simulink model "flightController"  (R2021a)
settings: Solver=ode3  StartTime=0  StopTime=TFinal  FixedStep=Ts  RelTol=1e-3  EnableMultiTasking=on
undefined symbols (not defined in the file): A, B, Controller, DiscIntNeverNeededParam, g, K, KLQI, KLQR, linsys, Ts, Vehicle
settings Model: Creator=The MathWorks, Inc.  LastModifiedBy=John
settings SolverCC: AlgebraicLoopSolver=TrustRegion  MinimalZcImpactIntegration=on
settings DataIOCC: LimitDataPoints=on  SaveFormat=Array  ReturnWorkspaceOutputs=off
settings OptimizationCC: BlockReduction=off  DefaultParameterBehavior=Inlined  BufferReuse=off  PassReuseOutputArgsThreshold=0
settings DebuggingCC: AlgebraicLoopMsg=none  ParameterPrecisionLossMsg=none  ParameterTunabilityLossMsg=error  UnconnectedInputMsg=none  UnconnectedOutputMsg=none  UnconnectedLineMsg=none  BusObjectLabelMismatch=error  SFUnexpectedBacktrackingDiag=warning  SFNoUnconditionalDefaultTransitionDiag=warning  SFExecutionAtInitializationDiag=none  SFMachineParentedDataDiag=warning  ArithmeticOperatorsInVariantConditions=warning
settings HardwareCC: ProdBitPerPointer=32  ProdBitPerSizeT=32  ProdBitPerPtrDiffT=32  ProdLargestAtomicInteger=Long  ProdWordSize=32  ProdHWDeviceType=ARM Compatible->ARM 9
settings ModelReferenceCC: ModelReferenceNumInstancesAllowed=Single  PropagateSignalLabelsOutOfModel=off
settings SFSimCC: SimUseLocalCustomCode=off  CustomCodeUndefinedFunction=UseInterfaceOnly
settings RTWCC: Description=Generic Real-Time Target  GenerateReport=on  RTWUseLocalCustomCode=off  LaunchReport=on
settings CodeAppCC: ForceParamTrailComments=on  MaxIdLength=63  OperatorAnnotations=on  StateflowObjectComments=on  MATLABSourceComments=on
settings GRTTargetCC: TargetLangStandard=C89/C90 (ANSI)
settings ConfigComp: CovMetricSettings=dw  CovSaveCumulativeToWorkspaceVar=on  CovSaveSingleToWorkspaceVar=on  CovExternalEMLEnable=off  CovSFcnEnable=off

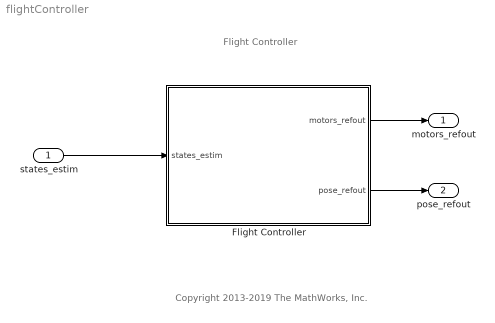
== system flightController ==
  note: Flight Controller
  note: Copyright 2013-2019 The MathWorks, Inc.
  states_estim : Inport  OutDataTypeStr=Bus: statesEstim_t  BusOutputAsStruct=on
  Flight Controller : Subsystem
  motors_refout : Outport  VectorParamsAs1DForOutWhenUnconnected=off
  pose_refout : Outport  Port=2  VectorParamsAs1DForOutWhenUnconnected=off
  wires:
  states_estim/1 -> Flight Controller/1(states_estim)
  Flight Controller/2(pose_refout) -> pose_refout/1
  Flight Controller/1(motors_refout) -> motors_refout/1

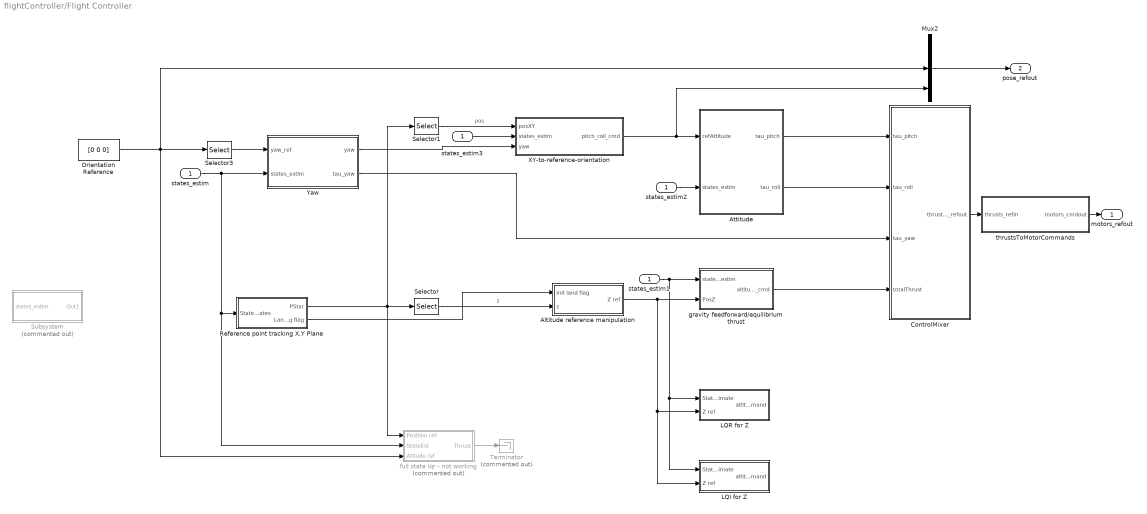
== system flightController/Flight Controller ==
  states_estim : Inport
  Altitude reference manipulation : Subsystem
  Attitude : Subsystem
  ControlMixer : Subsystem
  LQI for Z : Subsystem
  LQR for Z : Subsystem
  Mux2 : Mux  Inputs=3
  Orientation Reference : Constant  Value=[0 0 0]  OutDataTypeStr=single
  Reference point tracking X,Y Plane : Subsystem
  Selector : Selector  InputPortWidth=3  IndexOptions=Index vector (dialog)  Indices=3  OutputSizes=1
  Selector1 : Selector  InputPortWidth=3  IndexOptions=Index vector (dialog)  Indices=[1 2]  OutputSizes=1
  Selector3 : Selector  InputPortWidth=3  IndexOptions=Index vector (dialog)  Indices=1  OutputSizes=1
  Subsystem : Subsystem  Commented=on
  Terminator : Terminator  Commented=on
  XY-to-reference-orientation : Subsystem
  Yaw : Subsystem
  full state lqr - not working : Subsystem  Commented=on
  gravity feedforward/equilibrium thrust : Subsystem
  states_estim1 : InportShadow
  states_estim2 : InportShadow
  states_estim3 : InportShadow
  thrustsToMotorCommands : Subsystem
  motors_refout : Outport  VectorParamsAs1DForOutWhenUnconnected=off
  pose_refout : Outport  Port=2  VectorParamsAs1DForOutWhenUnconnected=off
  wires:
  thrustsToMotorCommands/1(motors_cmdout) -> motors_refout/1
  Selector3/1 -> Yaw/1(yaw_ref)
  Selector1/1 -> XY-to-reference-orientation/1(posXY)  "pos"
  ControlMixer/1(thrusts_refout) -> thrustsToMotorCommands/1(thrusts_refin)
  XY-to-reference-orientation/1(pitch_roll_cmd) -> Mux2/3, Attitude/1(refAttitude)
  Yaw/1(yaw) -> XY-to-reference-orientation/3(yaw)
  Mux2/1 -> pose_refout/1
  Attitude/1(tau_pitch) -> ControlMixer/1(tau_pitch)
  Attitude/2(tau_roll) -> ControlMixer/2(tau_roll)
  Yaw/2(tau_yaw) -> ControlMixer/3(tau_yaw)
  states_estim1/1 -> gravity feedforward/equilibrium thrust/1(states_estim), LQI for Z/1(State estimate), LQR for Z/1(State Estimate)
  states_estim2/1 -> Attitude/2(states_estim)
  states_estim3/1 -> XY-to-reference-orientation/2(states_estim)
  Orientation Reference/1 -> Selector3/1, Mux2/2, full state lqr - not working/3(Atitude ref)
  states_estim/1 -> full state lqr - not working/2(StateEst), Reference point tracking X,Y Plane/1(State estimates), Yaw/2(states_estim)
  Altitude reference manipulation/1(Z ref) -> LQI for Z/2(Z ref), LQR for Z/2(Z ref), gravity feedforward/equilibrium thrust/2(PosZ)
  Selector/1 -> Altitude reference manipulation/2(z)  "z"
  Reference point tracking X,Y Plane/2(Landing flag) -> Altitude reference manipulation/1(Init land flag)
  Reference point tracking X,Y Plane/1(PStar) -> full state lqr - not working/1(Position ref), Selector1/1, Selector/1
  full state lqr - not working/1(Thrust) -> Terminator/1
  gravity feedforward/equilibrium thrust/1(altitude_cmd) -> ControlMixer/4(totalThrust)

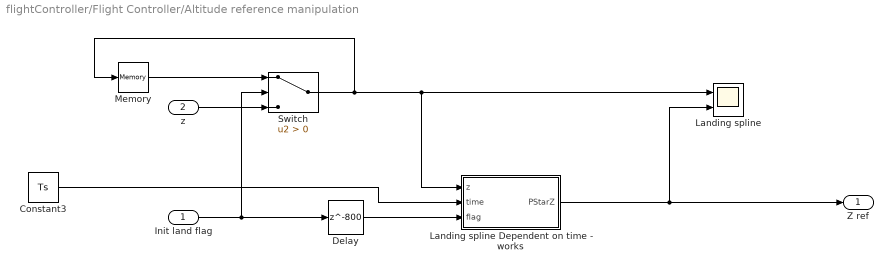
== system flightController/Flight Controller/Altitude reference manipulation ==
  Init land flag : Inport
  z : Inport  Port=2
  Constant3 : Constant  Value=Ts
  Delay : Delay  DelayLength=800
  Landing spline : Scope  NumInputPorts=2
  Landing spline Dependent on time - works : MATLAB Function  TreatAsAtomicUnit=on
  Memory : Memory
  Switch : Switch  Criteria=u2 > Threshold
  Z ref : Outport
  wires:
  Constant3/1 -> Landing spline Dependent on time - works/2(time)
  Delay/1 -> Landing spline Dependent on time - works/3(flag)
  Landing spline Dependent on time - works/1(PStarZ) -> Landing spline/2, Z ref/1
  Init land flag/1 -> Switch/2, Delay/1
  z/1 -> Switch/3
  Switch/1 -> Memory/1, Landing spline/1, Landing spline Dependent on time - works/1(z)
  Memory/1 -> Switch/1

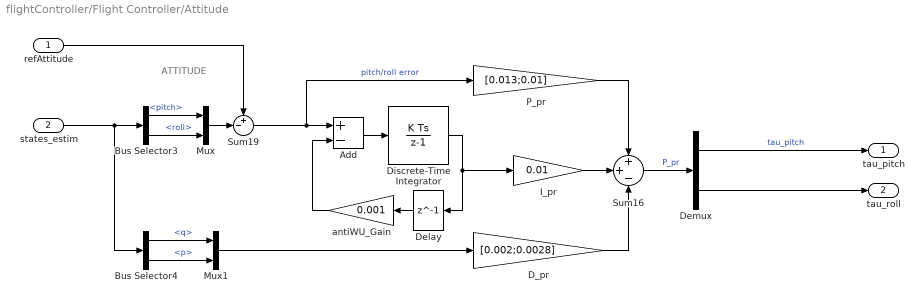
== system flightController/Flight Controller/Attitude ==
  note: ATTITUDE
  refAttitude : Inport
  states_estim : Inport  Port=2
  Add : Sum  Inputs=+-
  Bus Selector3 : BusSelector  OutputSignals=pitch,roll
  Bus Selector4 : BusSelector  OutputSignals=q,p
  D_pr : Gain  Gain=[0.002;0.0028]
  Delay : Delay  DelayLength=1  InitialCondition=0
  Demux : Demux  Outputs=2
  Discrete-Time Integrator : DiscreteIntegrator  SampleTime=Ts  LimitOutput=on  UpperSaturationLimit=2  LowerSaturationLimit=-2  ICPrevOutput=DiscIntNeverNeededParam  ICPrevScaledInput=DiscIntNeverNeededParam
  I_pr : Gain  Gain=0.01
  Mux : Mux  Inputs=2
  Mux1 : Mux  Inputs=2
  P_pr : Gain  Gain=[0.013;0.01]
  Sum16 : Sum  Inputs=++-  AccumDataTypeStr=single  OutDataTypeStr=single  SaturateOnIntegerOverflow=on
  Sum19 : Sum  Inputs=+-|
  antiWU_Gain : Gain  Gain=0.001
  tau_pitch : Outport  VectorParamsAs1DForOutWhenUnconnected=off
  tau_roll : Outport  Port=2  VectorParamsAs1DForOutWhenUnconnected=off
  wires:
  Sum16/1 -> Demux/1  "P_pr"
  antiWU_Gain/1 -> Add/2
  Add/1 -> Discrete-Time Integrator/1
  Bus Selector3/1 -> Mux/1  "<pitch>"
  Bus Selector4/1 -> Mux1/1  "<q>"
  P_pr/1 -> Sum16/1
  I_pr/1 -> Sum16/2
  Sum19/1 -> Add/1, P_pr/1  "pitch/roll error"
  Discrete-Time Integrator/1 -> Delay/1, I_pr/1
  Delay/1 -> antiWU_Gain/1
  Demux/1 -> tau_pitch/1  "tau_pitch"
  Demux/2 -> tau_roll/1
  D_pr/1 -> Sum16/3
  states_estim/1 -> Bus Selector3/1, Bus Selector4/1
  refAttitude/1 -> Sum19/1
  Mux/1 -> Sum19/2
  Bus Selector3/2 -> Mux/2  "<roll>"
  Mux1/1 -> D_pr/1
  Bus Selector4/2 -> Mux1/2  "<p>"

== system flightController/Flight Controller/ControlMixer ==
  tau_pitch : Inport
  tau_roll : Inport  Port=2
  tau_yaw : Inport  Port=3
  totalThrust : Inport  Port=4
  Mux2 : Mux
  Product : Product  Multiplication=Matrix(*)  RndMeth=Zero
  TorqueTotalThrustToThrustPerMotor : Constant  Value=Controller.Q2Ts  OutDataTypeStr=single
  thrusts_refout : Outport  VectorParamsAs1DForOutWhenUnconnected=off
  wires:
  Product/1 -> thrusts_refout/1
  tau_roll/1 -> Mux2/4
  tau_pitch/1 -> Mux2/3
  tau_yaw/1 -> Mux2/2
  totalThrust/1 -> Mux2/1
  TorqueTotalThrustToThrustPerMotor/1 -> Product/1
  Mux2/1 -> Product/2

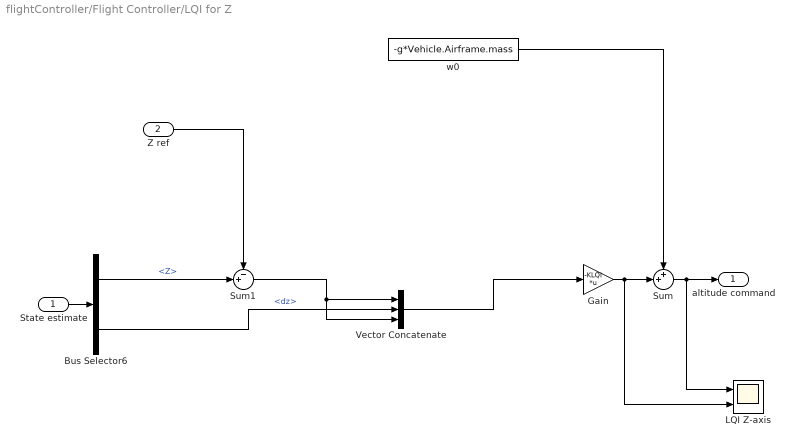
== system flightController/Flight Controller/LQI for Z ==
  State estimate : Inport
  Z ref : Inport  Port=2
  Bus Selector6 : BusSelector  OutputSignals=Z,dz
  Gain : Gain  Gain=-KLQI  Multiplication=Matrix(K*u) (u vector)
  LQI Z-axis : Scope  NumInputPorts=2
  Sum : Sum  Inputs=++|
  Sum1 : Sum  Inputs=-+|
  Vector Concatenate : Concatenate  NumInputs=3
  w0 : Constant  Value=-g*Vehicle.Airframe.mass  OutDataTypeStr=single  SampleTime=Ts
  altitude command : Outport
  wires:
  Bus Selector6/2 -> Vector Concatenate/2  "<dz>"
  State estimate/1 -> Bus Selector6/1
  Bus Selector6/1 -> Sum1/2  "<Z>"
  w0/1 -> Sum/1
  Gain/1 -> LQI Z-axis/2, Sum/2
  Sum/1 -> LQI Z-axis/1, altitude command/1
  Z ref/1 -> Sum1/1
  Sum1/1 -> Vector Concatenate/1, Vector Concatenate/3
  Vector Concatenate/1 -> Gain/1

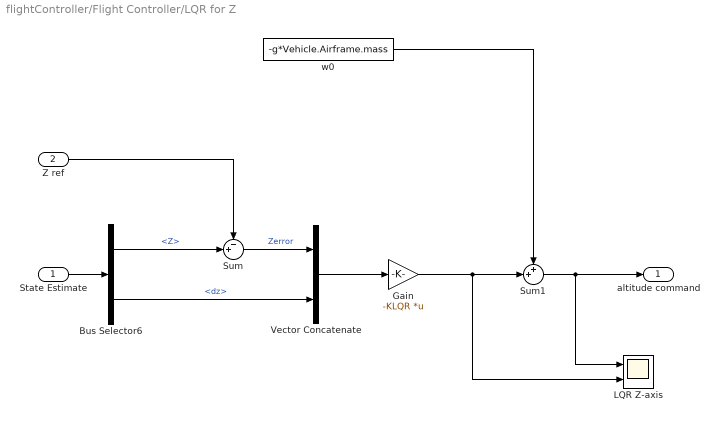
== system flightController/Flight Controller/LQR for Z ==
  State Estimate : Inport
  Z ref : Inport  Port=2
  Bus Selector6 : BusSelector  OutputSignals=Z,dz
  Gain : Gain  Gain=-KLQR  Multiplication=Matrix(K*u) (u vector)
  LQR Z-axis : Scope  NumInputPorts=2
  Sum : Sum  Inputs=-+|
  Sum1 : Sum  Inputs=++|
  Vector Concatenate : Concatenate
  w0 : Constant  Value=-g*Vehicle.Airframe.mass  OutDataTypeStr=single  SampleTime=Ts
  altitude command : Outport
  wires:
  Bus Selector6/2 -> Vector Concatenate/2  "<dz>"
  State Estimate/1 -> Bus Selector6/1
  Bus Selector6/1 -> Sum/2  "<Z>"
  Z ref/1 -> Sum/1
  Sum/1 -> Vector Concatenate/1  "Zerror"
  Vector Concatenate/1 -> Gain/1
  w0/1 -> Sum1/1
  Gain/1 -> LQR Z-axis/2, Sum1/2
  Sum1/1 -> LQR Z-axis/1, altitude command/1

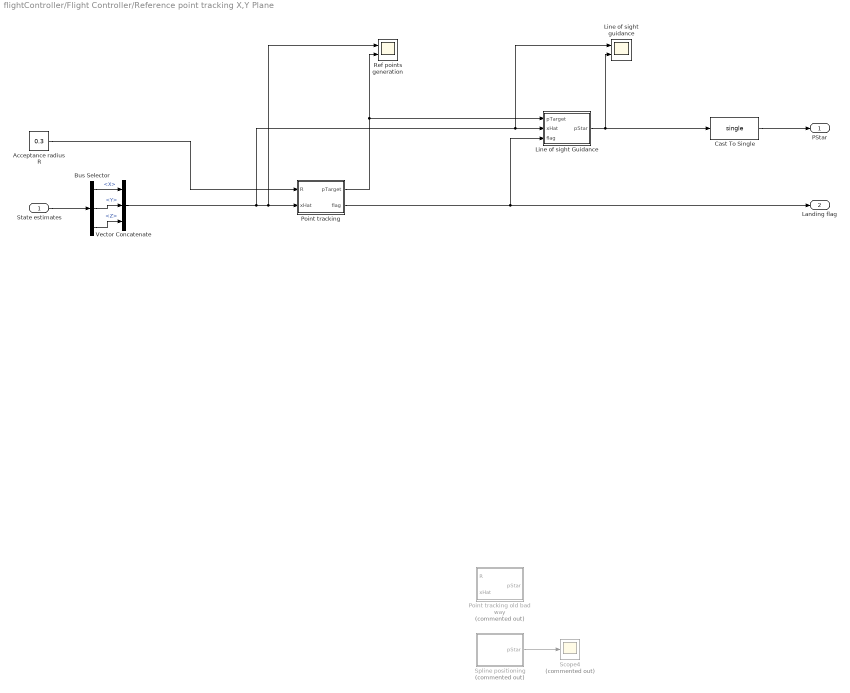
== system flightController/Flight Controller/Reference point tracking X,Y Plane ==
  State estimates : Inport
  Acceptance radius R : Constant  Value=0.3
  Bus Selector : BusSelector  OutputSignals=X,Y,Z
  Cast To Single : DataTypeConversion  OutDataTypeStr=single
  Line of sight Guidance : MATLAB Function  TreatAsAtomicUnit=on
  Line of sight guidance : Scope  NumInputPorts=2
  Point tracking : MATLAB Function  TreatAsAtomicUnit=on
  Point tracking old bad way : MATLAB Function  Commented=on  TreatAsAtomicUnit=on
  Ref points generation : Scope  NumInputPorts=2
  Scope4 : Scope  Commented=on
  Spline positioning : MATLAB Function  Commented=on  TreatAsAtomicUnit=on
  Vector Concatenate : Concatenate  NumInputs=3
  PStar : Outport
  Landing flag : Outport  Port=2
  wires:
  Bus Selector/3 -> Vector Concatenate/3  "<Z>"
  Bus Selector/1 -> Vector Concatenate/1  "<X>"
  Point tracking/1(pTarget) -> Line of sight Guidance/1(pTarget), Ref points generation/2
  Acceptance radius R/1 -> Point tracking/1(R)
  Bus Selector/2 -> Vector Concatenate/2  "<Y>"
  Vector Concatenate/1 -> Line of sight guidance/1, Line of sight Guidance/2(xHat), Ref points generation/1, Point tracking/2(xHat)
  Line of sight Guidance/1(pStar) -> Line of sight guidance/2, Cast To Single/1
  Point tracking/2(flag) -> Line of sight Guidance/3(flag), Landing flag/1
  State estimates/1 -> Bus Selector/1
  Cast To Single/1 -> PStar/1
  Spline positioning/1(pStar) -> Scope4/1

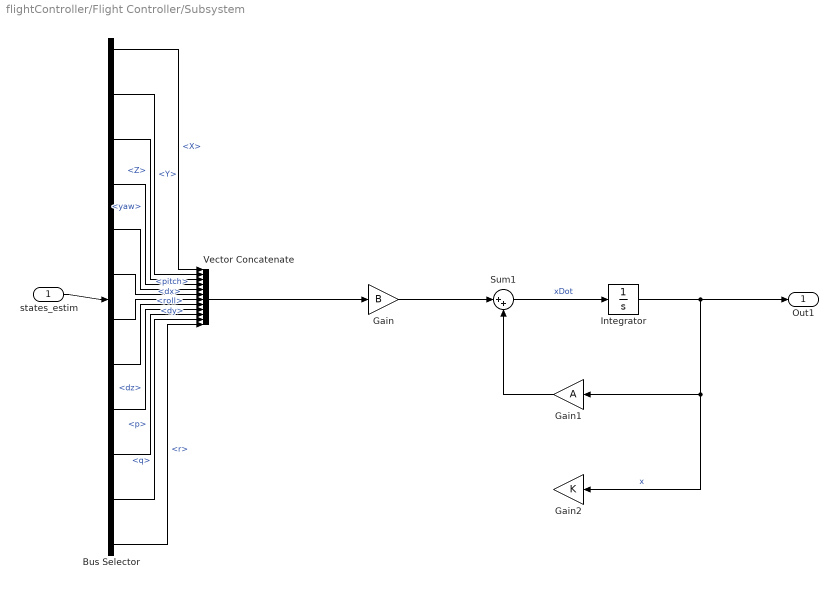
== system flightController/Flight Controller/Subsystem ==
  states_estim : Inport
  Bus Selector : BusSelector  OutputSignals=X,Y,Z,yaw,pitch,roll,dx,dy,dz,p,q,r
  Gain : Gain  Gain=B
  Gain1 : Gain  Gain=A
  Gain2 : Gain  Gain=K
  Integrator : Integrator
  Sum1 : Sum  Inputs=|++
  Vector Concatenate : Concatenate  NumInputs=12
  Out1 : Outport
  wires:
  Gain/1 -> Sum1/1
  Gain1/1 -> Sum1/2
  Sum1/1 -> Integrator/1  "xDot"
  Vector Concatenate/1 -> Gain/1
  Integrator/1 -> Gain1/1, Gain2/1, Out1/1  "x"
  states_estim/1 -> Bus Selector/1
  Bus Selector/1 -> Vector Concatenate/1  "<X>"
  Bus Selector/2 -> Vector Concatenate/2  "<Y>"
  Bus Selector/3 -> Vector Concatenate/3  "<Z>"
  Bus Selector/4 -> Vector Concatenate/4  "<yaw>"
  Bus Selector/5 -> Vector Concatenate/5  "<pitch>"
  Bus Selector/6 -> Vector Concatenate/6  "<roll>"
  Bus Selector/7 -> Vector Concatenate/7  "<dx>"
  Bus Selector/8 -> Vector Concatenate/8  "<dy>"
  Bus Selector/9 -> Vector Concatenate/9  "<dz>"
  Bus Selector/10 -> Vector Concatenate/10  "<p>"
  Bus Selector/11 -> Vector Concatenate/11  "<q>"
  Bus Selector/12 -> Vector Concatenate/12  "<r>"

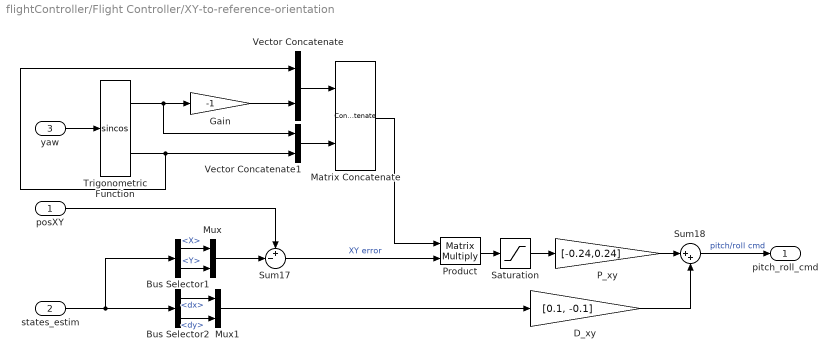
== system flightController/Flight Controller/XY-to-reference-orientation ==
  posXY : Inport
  states_estim : Inport  Port=2
  yaw : Inport  Port=3
  Bus Selector1 : BusSelector  OutputSignals=X,Y
  Bus Selector2 : BusSelector  OutputSignals=dx,dy
  D_xy : Gain  Gain=[0.1, -0.1]  ParamDataTypeStr=single  OutDataTypeStr=single  SaturateOnIntegerOverflow=on
  Gain : Gain  Gain=-1
  Matrix Concatenate : Concatenate  Mode=Multidimensional array  ConcatenateDimension=2
  Mux : Mux  Inputs=2
  Mux1 : Mux  Inputs=2
  P_xy : Gain  Gain=[-0.24,0.24]  ParamDataTypeStr=single  OutDataTypeStr=single  SaturateOnIntegerOverflow=on
  Product : Product  Multiplication=Matrix(*)  OutDataTypeStr=single  RndMeth=Zero
  Saturation : Saturate  UpperLimit=3  LowerLimit=-3  OutDataTypeStr=single
  Sum17 : Sum  Inputs=+-|  AccumDataTypeStr=single
  Sum18 : Sum  Inputs=|++  AccumDataTypeStr=single  OutDataTypeStr=single  SaturateOnIntegerOverflow=on
  Trigonometric Function : Trigonometry  Operator=sincos
  Vector Concatenate : Concatenate
  Vector Concatenate1 : Concatenate
  pitch_roll_cmd : Outport  VectorParamsAs1DForOutWhenUnconnected=off
  wires:
  yaw/1 -> Trigonometric Function/1
  Saturation/1 -> P_xy/1
  P_xy/1 -> Sum18/1
  Sum17/1 -> Product/2  "XY error"
  posXY/1 -> Sum17/1
  Bus Selector2/1 -> Mux1/1  "<dx>"
  states_estim/1 -> Bus Selector1/1, Bus Selector2/1
  Sum18/1 -> pitch_roll_cmd/1  "pitch/roll cmd"
  D_xy/1 -> Sum18/2
  Bus Selector1/1 -> Mux/1  "<X>"
  Product/1 -> Saturation/1
  Trigonometric Function/1 -> Gain/1, Vector Concatenate1/1
  Trigonometric Function/2 -> Vector Concatenate1/2, Vector Concatenate/1
  Gain/1 -> Vector Concatenate/2
  Vector Concatenate/1 -> Matrix Concatenate/1
  Vector Concatenate1/1 -> Matrix Concatenate/2
  Matrix Concatenate/1 -> Product/1
  Bus Selector1/2 -> Mux/2  "<Y>"
  Mux/1 -> Sum17/2
  Mux1/1 -> D_xy/1
  Bus Selector2/2 -> Mux1/2  "<dy>"

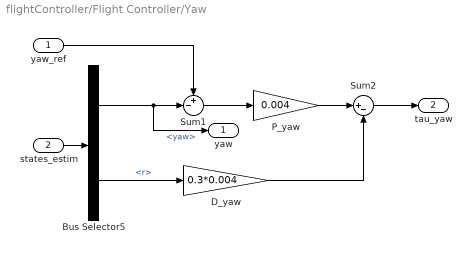
== system flightController/Flight Controller/Yaw ==
  yaw_ref : Inport
  states_estim : Inport  Port=2
  Bus Selector5 : BusSelector  OutputSignals=yaw,r
  D_yaw : Gain  Gain=0.3*0.004
  P_yaw : Gain  Gain=0.004  ParamDataTypeStr=single  OutDataTypeStr=single
  Sum1 : Sum  Inputs=+-|  AccumDataTypeStr=single  OutDataTypeStr=single  SaturateOnIntegerOverflow=on
  Sum2 : Sum  Inputs=|+-
  yaw : Outport  VectorParamsAs1DForOutWhenUnconnected=off
  tau_yaw : Outport  Port=2  VectorParamsAs1DForOutWhenUnconnected=off
  wires:
  D_yaw/1 -> Sum2/2
  P_yaw/1 -> Sum2/1
  Bus Selector5/2 -> D_yaw/1  "<r>"
  Sum1/1 -> P_yaw/1
  states_estim/1 -> Bus Selector5/1
  Sum2/1 -> tau_yaw/1
  Bus Selector5/1 -> yaw/1, Sum1/2  "<yaw>"
  yaw_ref/1 -> Sum1/1

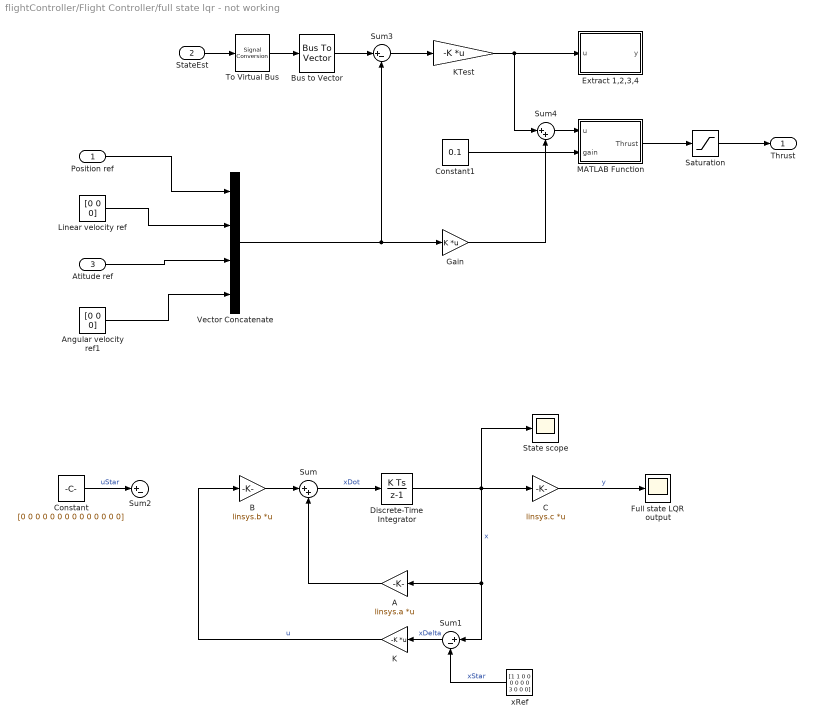
== system flightController/Flight Controller/full state lqr - not working ==
  Position ref : Inport
  StateEst : Inport  Port=2
  Atitude ref : Inport  Port=3
  A : Gain  Gain=linsys.a  Multiplication=Matrix(K*u) (u vector)
  Angular velocity ref1 : Constant  Value=[0 0 0]  OutDataTypeStr=single
  B : Gain  Gain=linsys.b  Multiplication=Matrix(K*u) (u vector)
  Bus to Vector : BusToVector
  C : Gain  Gain=linsys.c  Multiplication=Matrix(K*u) (u vector)
  Constant : Constant  Value=[0 0 0 0 0 0 0 0 0 0 0 0 0 0]
  Constant1 : Constant  Value=0.1
  Discrete-Time Integrator : DiscreteIntegrator  InitialCondition=[0 0 0 0 0 0 0 0 0 0 0 0]  SampleTime=-1  ICPrevOutput=DiscIntNeverNeededParam  ICPrevScaledInput=DiscIntNeverNeededParam
  Extract 1,2,3,4 : MATLAB Function  TreatAsAtomicUnit=on
  Full state LQR output : Scope
  Gain : Gain  Gain=K  Multiplication=Matrix(K*u) (u vector)
  K : Gain  Gain=-K  Multiplication=Matrix(K*u) (u vector)
  KTest : Gain  Gain=-K  Multiplication=Matrix(K*u) (u vector)
  Linear velocity ref : Constant  Value=[0 0 0]  OutDataTypeStr=single
  MATLAB Function : MATLAB Function  TreatAsAtomicUnit=on
  Saturation : Saturate  UpperLimit=1  LowerLimit=-1
  State scope : Scope
  Sum : Sum  Inputs=|++
  Sum1 : Sum  Inputs=|+-
  Sum2 : Sum  Inputs=|+-
  Sum3 : Sum  Inputs=|+-
  Sum4 : Sum  Inputs=|++
  To Virtual Bus : SignalConversion  ConversionOutput=Virtual bus  OverrideOpt=off
  Vector Concatenate : Concatenate  NumInputs=4
  xRef : Constant  Value=[1 1 0 0 0 0 0 0 3 0 0 0]
  Thrust : Outport
  wires:
  StateEst/1 -> To Virtual Bus/1
  To Virtual Bus/1 -> Bus to Vector/1
  B/1 -> Sum/1
  A/1 -> Sum/2
  Sum/1 -> Discrete-Time Integrator/1  "xDot"
  Discrete-Time Integrator/1 -> State scope/1, A/1, Sum1/1, C/1  "x"
  K/1 -> B/1  "u"
  Sum1/1 -> K/1  "xDelta"
  xRef/1 -> Sum1/2  "xStar"
  Constant/1 -> Sum2/1  "uStar"
  C/1 -> Full state LQR output/1  "y"
  Bus to Vector/1 -> Sum3/1
  Sum3/1 -> KTest/1
  Position ref/1 -> Vector Concatenate/1
  Linear velocity ref/1 -> Vector Concatenate/2
  Atitude ref/1 -> Vector Concatenate/3
  Angular velocity ref1/1 -> Vector Concatenate/4
  Vector Concatenate/1 -> Gain/1, Sum3/2
  Constant1/1 -> MATLAB Function/2(gain)
  Sum4/1 -> MATLAB Function/1(u)
  KTest/1 -> Sum4/1, Extract 1,2,3,4/1(u)
  MATLAB Function/1(Thrust) -> Saturation/1
  Saturation/1 -> Thrust/1
  Gain/1 -> Sum4/2

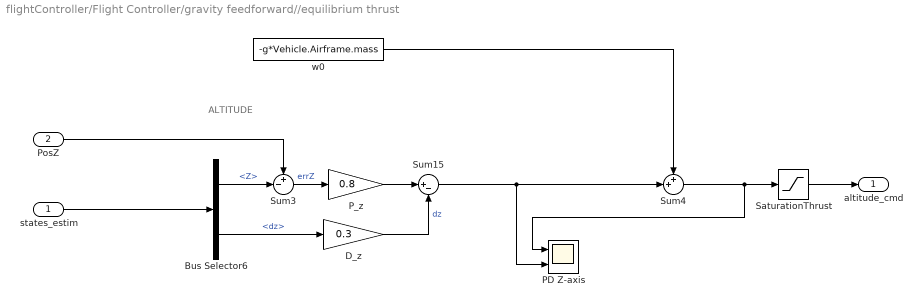
== system flightController/Flight Controller/gravity feedforward//equilibrium thrust ==
  note: ALTITUDE
  states_estim : Inport
  PosZ : Inport  Port=2
  Bus Selector6 : BusSelector  OutputSignals=Z,dz
  D_z : Gain  Gain=0.3  ParamDataTypeStr=single  OutDataTypeStr=single  SaturateOnIntegerOverflow=on
  PD Z-axis : Scope  NumInputPorts=2
  P_z : Gain  Gain=0.8  ParamDataTypeStr=single  OutDataTypeStr=single  SaturateOnIntegerOverflow=on
  SaturationThrust : Saturate  UpperLimit=4*Controller.totalThrustMaxRelative*Controller.motorsThrustPerMotorMax  LowerLimit=-4*Controller.totalThrustMaxRelative*Controller.motorsThrustPerMotorMax  OutDataTypeStr=single
  Sum15 : Sum  Inputs=|+-  AccumDataTypeStr=single  OutDataTypeStr=single  SaturateOnIntegerOverflow=on
  Sum3 : Sum  Inputs=+-|  AccumDataTypeStr=single  OutDataTypeStr=single  SaturateOnIntegerOverflow=on
  Sum4 : Sum  Inputs=++|  AccumDataTypeStr=single  OutDataTypeStr=single  SaturateOnIntegerOverflow=on
  w0 : Constant  Value=-g*Vehicle.Airframe.mass  OutDataTypeStr=single  SampleTime=Ts
  altitude_cmd : Outport  VectorParamsAs1DForOutWhenUnconnected=off
  wires:
  Sum3/1 -> P_z/1  "errZ"
  Bus Selector6/1 -> Sum3/2  "<Z>"
  Bus Selector6/2 -> D_z/1  "<dz>"
  w0/1 -> Sum4/1
  D_z/1 -> Sum15/2  "dz"
  PosZ/1 -> Sum3/1
  P_z/1 -> Sum15/1
  Sum15/1 -> PD Z-axis/2, Sum4/2
  Sum4/1 -> PD Z-axis/1, SaturationThrust/1
  SaturationThrust/1 -> altitude_cmd/1
  states_estim/1 -> Bus Selector6/1

== system flightController/Flight Controller/thrustsToMotorCommands ==
  thrusts_refin : Inport
  MotorDirections : Gain  Gain=[1 -1 1 -1]
  Saturation5 : Saturate  UpperLimit=Vehicle.Motor.maxLimit  LowerLimit=Vehicle.Motor.minLimit
  ThrustToMotorCommand : Gain  Gain=-Vehicle.Motor.thrustToMotorCommand
  motors_cmdout : Outport  VectorParamsAs1DForOutWhenUnconnected=off
  wires:
  Saturation5/1 -> MotorDirections/1
  MotorDirections/1 -> motors_cmdout/1
  ThrustToMotorCommand/1 -> Saturation5/1
  thrusts_refin/1 -> ThrustToMotorCommand/1

== matlab function flightController/Flight Controller/Reference point tracking X,Y Plane/Spline positioning ==
  data: pStar output
function pStar = fcn()
xConstraints = [0 0 0.5 1 0.5 1 1.5 0];
yConstraints = [0 0 1   2 1   2 2   0];

persistent td;
if(isempty(td))
    td = 0;
end
td = td + 1;

sigma = 0;
b0 = [1 sigma sigma^2 sigma^3];
b0p = [0 1 2*sigma 3*sigma^2];

sigma = 10;
b1 = [1 sigma sigma^2 sigma^3];
b1pp = [0 0 2 6*sigma];

sigma = 20;
b2 = [1 sigma sigma^2 sigma^3];
b2p = [0 1 2*sigma 3*sigma^2];

BMat = [    b0   zeros(1,4);
            b0p  zeros(1,4);
            b1   zeros(1,4);
            b1pp zeros(1,4);
            zeros(1,4)   b1;
            zeros(1,4) b1pp;
            zeros(1,4)   b2;
            zeros(1,4)  b2p     ];
x = 0;
y = 0;
xAlpha = inv(BMat)*xConstraints';
yAlpha = inv(BMat)*yConstraints';

if(td <=10)
   x = xAlpha(1:4)'*[1 td td^2 td^3]';
   y = yAlpha(1:4)'*[1 td td^2 td^3]';
end
if(td > 10)
   x = xAlpha(5:8)'*[1 td td^2 td^3]';
   y = yAlpha(5:8)'*[1 td td^2 td^3]';
end

pStar = [x y -0.7]';

== matlab function flightController/Flight Controller/full state lqr - not working/Extract 1,2,3,4 ==
  data: u input; y output
function y = fcn(u)

y = u(1:4);

== matlab function flightController/Flight Controller/Reference point tracking X,Y Plane/Line of sight Guidance ==
  data: pTarget input; pStar output; xHat input; flag input
function pStar = fcn(pTarget, xHat, flag)
% This function generates small intermediate points between the actual position
% and the desired reference point, so that the controller will not be
% overwelmed by having to make a too large motor command that the drone
% cannot take without falling out of the skies.

% Initialize variables
%PxTilte = 0;
%PyTilte = 0;
k = 0.1;

% Calculate position error pTilte
PxTilte = xHat(1)-pTarget(1);
PyTilte = xHat(2)-pTarget(2);

% Calculate pTilte norm
pTilteNorm = sqrt(PxTilte^2+PyTilte^2);

% Velocity in the direction I want from pTiltes
vd_x = -k*(PxTilte/(pTilteNorm));
vd_y = -k*(PyTilte/(pTilteNorm));

if(flag == true)
    vd_x = single(0);
    vd_y = single(0);
end

pStar = [xHat(1)+vd_x xHat(2)+vd_y pTarget(3)]';


% The velocity constantly changes when hovering at a waypoint. 
% This will make the drone oscillate around that point.
% To stop this, the velocity calculation should stop when hovering

== matlab function flightController/Flight Controller/Reference point tracking X,Y Plane/Point tracking ==
  data: R input; pTarget output; xHat input; flag output
function [pTarget, flag]= fcn(R, xHat)
%% This function is only responsible for changing reference point when the 
% drone is within some radius R to the reference point. 
persistent i;
if(isempty(i))
    i = 1;
end
persistent temp;
if(isempty(temp))
    temp = false;
end
wayPoints = [0 0 -0.7; 1 0 -0.7; 0 1 -0.7; -1 0 -0.7];
if( R^2 >= ((xHat(1)-wayPoints(i,1))^2+(xHat(2)-wayPoints(i,2))^2) )
        i = i+1;
        if(i > length(wayPoints))
            i = length(wayPoints);
            temp = true;
        end
end
pTarget = wayPoints(i,:)';
flag = temp;

== matlab function flightController/Flight Controller/full state lqr - not working/MATLAB Function ==
  data: u input; Thrust output; gain input
function Thrust = fcn(u, gain)

Thrust = (((-u(1)-u(2)-u(3)-u(4))*1)*gain);

== matlab function flightController/Flight Controller/Altitude reference manipulation/Landing spline Dependent on time - works ==
  data: z input; PStarZ output; time input; flag input
function PStarZ= fcn(z, time, flag)
    zLanded = -0.011;
    zContraints = [z 0 zLanded 0]';
    t = 0;
    B0 = [1 t, t^2 t^3];
    BPrime0 = [0 1 2*t 3*t^2];
    
    t = 10;
    B1 = [1 t, t^2 t^3];
    BPrime1 = [0 1 2*t 3*t^2];

    BMat = [    B0;
                BPrime0;
                B1;
                BPrime1     ];
            
    Alpha = inv(BMat)*zContraints;
    
    persistent landed;
    if(isempty(landed))
        landed = 0;
    end
    persistent td;
    if(isempty(td))
       td = 0;
    end
    
    if(flag == true)
        td = td + time;
        P = Alpha'*[1 td td^2 td^3]';
        if(P >= zLanded)
            landed = 1;
        end
        if(landed == 1)
            P = single(zLanded);
        end
    else
        P = z;
    end
PStarZ = P;

== matlab function flightController/Flight Controller/Reference point tracking X,Y Plane/Point tracking old bad way ==
  data: R input; pStar output; xHat input
function pStar = fcn(R, xHat)
persistent i;
persistent td;
if(isempty(i))
    i = 1;
    td = 0;
end
td = td +1;
wayPoints = [0 0 -0.7; 1 0 -0.7; 0 1 -0.7; -1 0 -0.7; 0 -1 -0.7];
if( R^2 >= ((xHat(1)-wayPoints(i,1))^2+(xHat(2)-wayPoints(i,2)^2)) )
    if(td > 1000)
        i = i+1;
        td = 0;
        if(i > length(wayPoints))
            i = length(wayPoints);
        end
    end
end

pStar = wayPoints(i,:)';
